simulink model "H_inf_2020"  (R2020b)
settings: Solver=VariableStepAuto  StartTime=0.0  StopTime=10.0  RelTol=1e-3
values from neighbouring files (symbols this model uses):
  Ask = [0 1 0 0 ... (first row only)    [H_inf_ctrl.m]    (also in H_inf_ctrl_11_2.m; H_inf_ctrl_11_2_m.m)
  Bsk = [0 0 0 0 ... (first row only)    [H_inf_ctrl.m]    (also in H_inf_ctrl_11_2.m; H_inf_ctrl_11_2_m.m)
  Csk = [0 1 0 0 ... (first row only)    [H_inf_ctrl.m]    (also in H_inf_ctrl_11_2.m; H_inf_ctrl_11_2_m.m)
  Dsk = zeros(2,4)    [H_inf_ctrl.m]    (also in H_inf_ctrl_11_2.m; H_inf_ctrl_11_2_m.m)
undefined symbols (not defined in the file or in its folder): Ainf, Binf, Cinf, Dinf, sigbuilder_block
settings Model: Creator=tawsiful  LastModifiedBy=tawsiful
settings DebuggingCC: UnconnectedInputMsg=none  UnconnectedOutputMsg=none  UnconnectedLineMsg=none  SFMachineParentedDataDiag=error

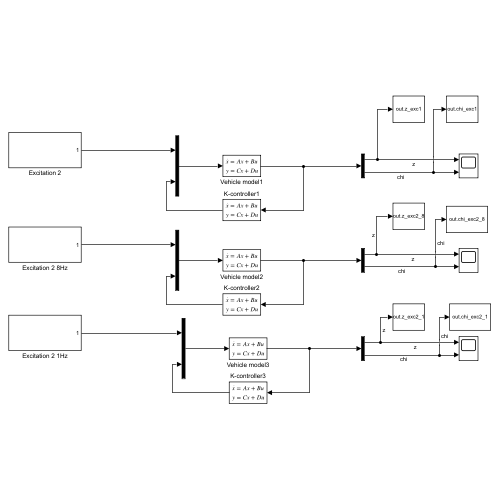
[thumbnail: Simulink's stored preview of the top-level diagram]
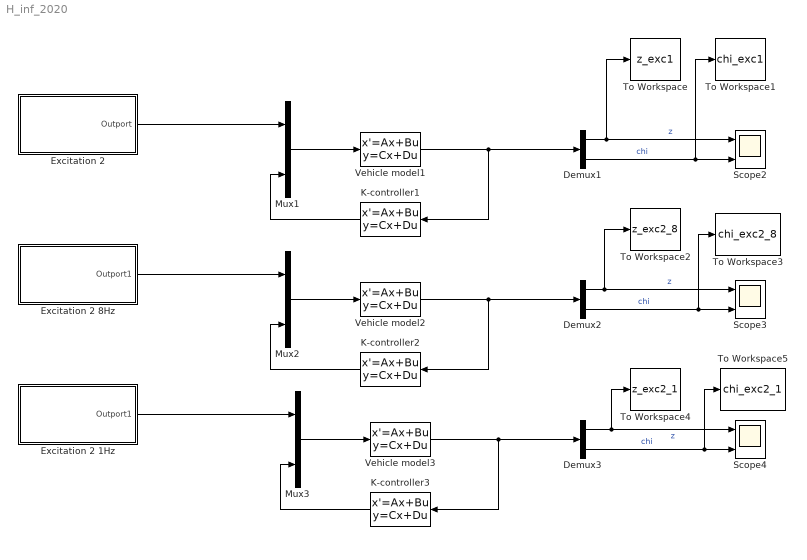
== system H_inf_2020 ==
  Demux1 : Demux  Outputs=2
  Demux2 : Demux  Outputs=2
  Demux3 : Demux  Outputs=2
  Excitation 2 : Subsystem
  Excitation 2 1Hz : Subsystem
  Excitation 2 8Hz : Subsystem
  K-controller1 : StateSpace  A=Ainf  B=Binf  C=Cinf  D=Dinf  InitialCondition=0
  K-controller2 : StateSpace  A=Ainf  B=Binf  C=Cinf  D=Dinf  InitialCondition=0
  K-controller3 : StateSpace  A=Ainf  B=Binf  C=Cinf  D=Dinf  InitialCondition=0
  Mux1 : Mux  Inputs=2
  Mux2 : Mux  Inputs=2
  Mux3 : Mux  Inputs=2
  Scope2 : Scope  NumInputPorts=2
  Scope3 : Scope  NumInputPorts=2
  Scope4 : Scope  NumInputPorts=2
  To Workspace : ToWorkspace  VariableName=z_exc1  SampleTime=-1
      settings: Save2DSignal=2-D array (concatenate along first dimension)
  To Workspace1 : ToWorkspace  VariableName=chi_exc1  SampleTime=-1
      settings: Save2DSignal=2-D array (concatenate along first dimension)
  To Workspace2 : ToWorkspace  VariableName=z_exc2_8  SampleTime=-1
      settings: Save2DSignal=2-D array (concatenate along first dimension)
  To Workspace3 : ToWorkspace  VariableName=chi_exc2_8  SampleTime=-1
      settings: Save2DSignal=2-D array (concatenate along first dimension)
  To Workspace4 : ToWorkspace  VariableName=z_exc2_1  SampleTime=-1
      settings: Save2DSignal=2-D array (concatenate along first dimension)
  To Workspace5 : ToWorkspace  VariableName=chi_exc2_1  SampleTime=-1
      settings: Save2DSignal=2-D array (concatenate along first dimension)
  Vehicle model1 : StateSpace  A=Ask  B=Bsk  C=Csk  D=Dsk  InitialCondition=0
  Vehicle model2 : StateSpace  A=Ask  B=Bsk  C=Csk  D=Dsk  InitialCondition=0
  Vehicle model3 : StateSpace  A=Ask  B=Bsk  C=Csk  D=Dsk  InitialCondition=0
  wires:
  Demux3/1 -> To Workspace4/1, Scope4/1  "z"
  Demux3/2 -> To Workspace5/1, Scope4/2  "chi"
  Demux1/2 -> To Workspace1/1, Scope2/2  "chi"
  Demux2/2 -> To Workspace3/1, Scope3/2  "chi"
  Demux1/1 -> Scope2/1, To Workspace/1  "z"
  Demux2/1 -> To Workspace2/1, Scope3/1  "z"
  Mux1/1 -> Vehicle model1/1
  Vehicle model1/1 -> Demux1/1, K-controller1/1
  K-controller1/1 -> Mux1/2
  K-controller2/1 -> Mux2/2
  Vehicle model2/1 -> Demux2/1, K-controller2/1
  Mux2/1 -> Vehicle model2/1
  Mux3/1 -> Vehicle model3/1
  Vehicle model3/1 -> Demux3/1, K-controller3/1
  K-controller3/1 -> Mux3/2
  Excitation 2/1(Outport) -> Mux1/1
  Excitation 2 8Hz/1(Outport1) -> Mux2/1
  Excitation 2 1Hz/1(Outport1) -> Mux3/1

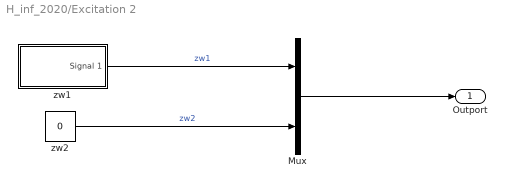
== system H_inf_2020/Excitation 2 ==
  Mux : Mux  Inputs=2
  zw1 : Subsystem  Tag=STV Subsys  LoadFcn=sigbuilder_block('load');  StartFcn=sigbuilder_block('start');  StopFcn=sigbuilder_block('stop');  ClipboardFcn=sigbuilder_block('clipboard');  mask(Sigbuilder block){tuvar=[0:10]}
      mask help: Simulink:masks:SigbuilderBlock_MD
      mask init:
      | if ~strcmp(get_param(bdroot(gcbh),'SimulationStatus'),'stopped') tuvar = sigbuilder_block('maskInit'); end
      settings: CopyFcn=sigbuilder_block('copy');  DeleteFcn=sigbuilder_block('delete');  ModelCloseFcn=sigbuilder_block('modelClose');  PreSaveFcn=sigbuilder_block('preSave');  PauseFcn=sigbuilder_block('pause');  ContinueFcn=sigbuilder_block('continue');  NameChangeFcn=sigbuilder_block('namechange');  OpenFcn=sigbuilder_block('open',[437.6 199.2 550.4 400 ]);  CloseFcn=sigbuilder_block('close');
      mask Display: plot(0, 0, 100, 100,[2, 2, 32, 32, 2], [68, 8, 8, 68, 68],[32, 2], [38, 38], [32, 19, 2],[53, 60, 44], [32, 17, 17, 2],[16, 16, 31, 31]);txt = getActiveGroup(gcbh);text(2, 100, txt,'verticalAlignment', 'top');
  zw2 : Constant  Value=0
  Outport : Outport
  wires:
  zw1/1(Signal 1) -> Mux/1  "zw1"
  zw2/1 -> Mux/2  "zw2"
  Mux/1 -> Outport/1

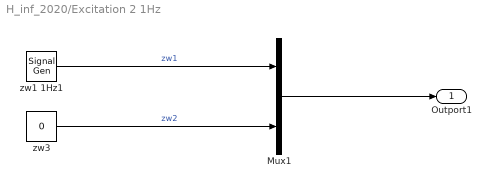
== system H_inf_2020/Excitation 2 1Hz ==
  Mux1 : Mux  Inputs=2
  zw1 1Hz1 : SignalGenerator  Amplitude=0.01  Frequency=2*pi*1  Units=rad/sec
  zw3 : Constant  Value=0
  Outport1 : Outport
  wires:
  zw3/1 -> Mux1/2  "zw2"
  zw1 1Hz1/1 -> Mux1/1  "zw1"
  Mux1/1 -> Outport1/1

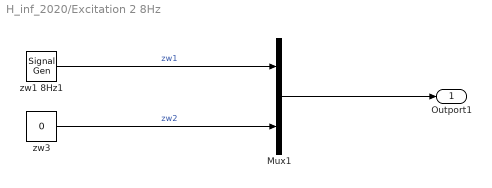
== system H_inf_2020/Excitation 2 8Hz ==
  Mux1 : Mux  Inputs=2
  zw1 8Hz1 : SignalGenerator  Amplitude=0.01  Frequency=2*pi*8  Units=rad/sec
  zw3 : Constant  Value=0
  Outport1 : Outport
  wires:
  zw3/1 -> Mux1/2  "zw2"
  zw1 8Hz1/1 -> Mux1/1  "zw1"
  Mux1/1 -> Outport1/1

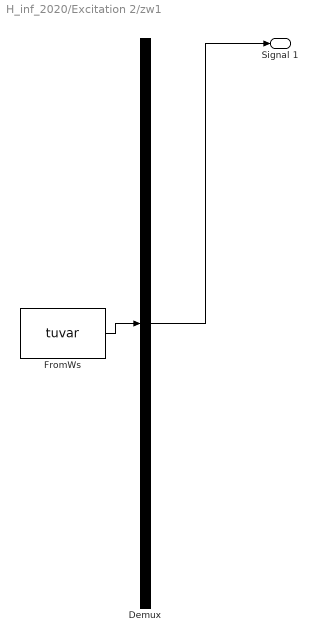
== system H_inf_2020/Excitation 2/zw1 ==
  Demux : Demux  Tag=STV Demux  Outputs=1
      settings: DisplayOption=none
  FromWs : FromWorkspace  Tag=STV FromWs  VariableName=tuvar
      SigBuilderData=|
      | common.afterFinalStr = 'Extrapolate'
      | common.sampleTime = 0
      | dataSet.timeRange = [0 10]
      | dataSet.name = 'Group 1'
      | sbobj.Groups.Name = 'Group 1'
      | sbobj.Groups.Signals.Name = 'Signal 1'
      | sbobj.Groups.Signals.XData = [0 0.1 0.1 10]
      | sbobj.Groups.Signals.YData = [0.03 0.03 0 0]
  Signal 1 : Outport  Tag=STV Outport
  wires:
  Demux/1 -> Signal 1/1
  FromWs/1 -> Demux/1
